simulink model "joystick2"  (R2020a)
settings: Solver=VariableStepAuto  StartTime=0.0  StopTime=inf  RelTol=1e-3
libraries: vrlib x1
settings Model: EnablePacing=on  Creator=john  LastModifiedBy=jhtran

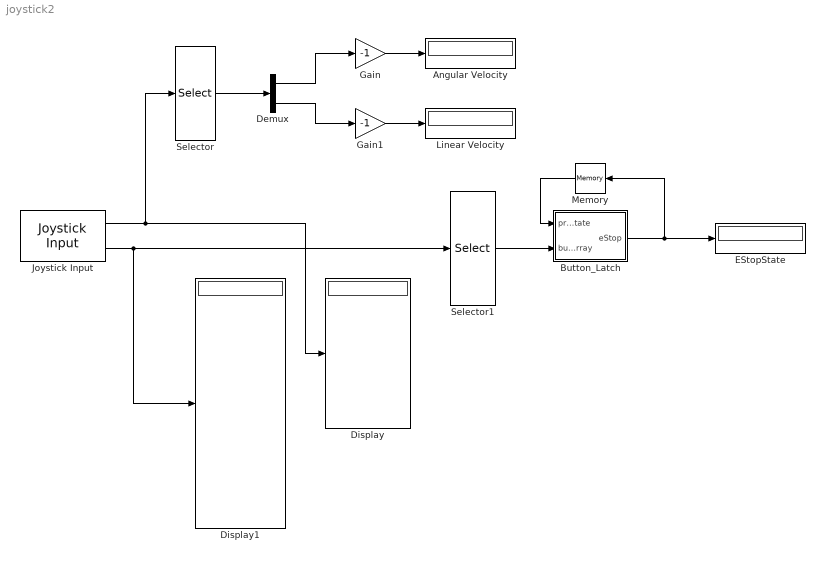
== system joystick2 ==
  Angular Velocity : Display
  Button_Latch : MATLAB Function  TreatAsAtomicUnit=on
  Demux : Demux  Outputs=2
  Display : Display
  Display1 : Display
  EStopState : Display
  Gain : Gain  Gain=-1
  Gain1 : Gain  Gain=-1
  Joystick Input : vrlib/Joystick Input  joyid=1  adjustports=on  forcefeed=on
  Linear Velocity : Display
  Memory : Memory
  Selector : Selector  InputPortWidth=8  IndexOptions=Index vector (dialog)  Indices=[1 2]  OutputSizes=1
  Selector1 : Selector  InputPortWidth=13  IndexOptions=Index vector (dialog)  Indices=[1 3]  OutputSizes=1
  wires:
  Joystick Input/1 -> Selector/1, Display/1
  Joystick Input/2 -> Display1/1, Selector1/1
  Selector/1 -> Demux/1
  Demux/1 -> Gain/1
  Gain/1 -> Angular Velocity/1
  Demux/2 -> Gain1/1
  Gain1/1 -> Linear Velocity/1
  Selector1/1 -> Button_Latch/2(buttonArray)
  Button_Latch/1(eStop) -> EStopState/1, Memory/1
  Memory/1 -> Button_Latch/1(prevEState)

== matlab function joystick2/Button_Latch ==
  data: prevEState input; buttonArray input; eStop output
function eStop = fcn(prevEState, buttonArray)

    % Copy previous E State
    currentEState = prevEState; 

    % Map Button Array
    eStopButton = buttonArray(1,1); 
    resetStopButton = buttonArray(2,1); 

    % Check if emergency button is pressed and st
    if eStopButton == 1 && currentEState == 0 
        
        % Set stop state to be 1
        currentEState = 1;
        
    % Check if reset button is pressed
    elseif resetStopButton == 1 && currentEState == 1
        
        % Set stop state to be 0 
        currentEState = 0; 
        
    end

eStop = currentEState;
